simulink model "ACC"  (R2013a)
settings: Solver=ode4  StartTime=0.0  StopTime=100  FixedStep=0.001  MaxStep=0.001  RelTol=1e-3
model workspace (MAT data in the model file):
  m = 1530
  lf = 1.11
  lr = 1.6662
  R_Tire = 0.33
  Iyy_Tire = 0.9
  Pb2Tq_f = 300
  Pb2Tq_r = 150
  Fx_SL = [-1; -0.9; -0.8; -0.7; -0.6; -0.5; -0.4; -0.3; -0.25; -0.2; -0.18; -0.16; -0.14; -0.12; -0.1; -0.08; -0.06; -0.04; -0.02; 0; 0.02; 0.04; 0.06; 0.08; 0.1; 0.12; 0.14; 0.16; 0.18; 0.2; 0.25; 0.3; 0.4; 0.5; 0.6; 0.7; 0.8; 0.9; 1]
  Fx_W = [2105 3995 6120 7900 10100]
  Fx_Data = [-2029.26  -4058.51  -6087.76  -8117.01  -10146.3; -2029.26  -4058.51  -6087.76  -8117.01  -10146.3; -2053.55  -4107.12  -6160.67  -8214.24  -10267.8; -2084.58  -4169.16  -6253.75  -8338.33  -10422.9; -2125.47  -4250.95  -6376.42  -8501.91  -10627.4; -2181.64  -4363.28  -6544.93  -8726.56  -10908.2; -2262.94  -4525.87  -6788.82  -9051.76  -11314.7; -2388.22  -4776.46  -7164.69  -9552.92  -11941.1; -2476.95  -4953.9  -7430.85  -9907.79  -12384.7; -2586.89  -5173.78  -7760.68  -10347.6  -12934.4; -2634.75  -5269.5  -7904.24  -10539  -13173.7; -2680.7  -5361.4  -8042.1  -10722.8  -13403.5; -2717.36  -5434.73  -8152.09  -10869.4  -13586.8; -2729.82  -5459.63  -8189.45  -10919.3  -13649.1; -2689.78  -5379.54  -8069.32  -10759.1  -13448.8; -2548.95  -5097.92  -7646.88  -10195.8  -12744.8; -2240.07  -4480.13  -6720.21  -8960.27  -11200.3; -1701.43  -3402.86  -5104.29  -6805.72  -8507.15; -926.741  -1853.48  -2780.22  -3706.97  -4633.7; 0  0  0  0  0; 926.741  1853.48  2780.22  3706.97  4633.7; 1701.43  3402.86  5104.29  6805.72  8507.15; 2240.07  4480.13  6720.21  8960.27  11200.3; 2548.95  5097.92  7646.88  10195.8  12744.8; 2689.78  5379.54  8069.32  10759.1  13448.8; 2729.82  5459.63  8189.45  10919.3  13649.1; 2717.36  5434.73  8152.09  10869.4  13586.8; 2680.7  5361.4  8042.1  10722.8  13403.5; 2634.75  5269.5  7904.24  10539  13173.7; 2586.89  5173.78  7760.68  10347.6  12934.4; 2476.95  4953.9  7430.85  9907.79  12384.7; 2388.22  4776.46  7164.69  9552.92  11941.1; 2262.94  4525.87  6788.82  9051.76  11314.7; 2181.64  4363.28  6544.93  8726.56  10908.2; 2125.47  4250.95  6376.42  8501.91  10627.4; 2084.58  4169.16  6253.75  8338.33  10422.9; 2053.55  4107.12  6160.67  8214.24  10267.8; 2029.26  4058.51  6087.76  8117.01  10146.3; 2029.26  4058.51  6087.76  8117.01  10146.3]
  g = 9.81
  t2e = 2000
  Fy_Angle = [-20; -16; -14; -12; -10; -9.5; -9; -8.5; -8; -7.5; -7; -6.5; -6; -5.5; -5; -4.5; -4; -3.5; -3; -2.5; -2; -1.5; -1; -0.5; 0; 0.5; 1; 1.5; 2; 2.5; 3; 3.5; 4; 4.5; 5; 5.5; 6; 6.5; 7; 7.5; 8; 8.5; 9; 9.5; 10; 12; 14; 16; 18; 20]
  Fy_W = [1725 3500 6100 6950 9005]
  Fy_Data = [-1523.64 -1531.91 -1546.58 -1574.53 -1631.62 -1653.27 -1678.67 -1707.8 -1740.18 -1775.12 -1810.95 -1845.3 ... (250 elements, 50x5)]
  Cr = 38255
  Cf = 38925
  Izz = 4192
  GearRatio = 17.25
  K = 19
  mu = 0.9
undefined symbols (not defined in the file): sigbuilder_block
libraries: simulink x3
settings Model: Creator=Park  LastModifiedBy=IVDL
settings DataIOCC: LimitDataPoints=off  SignalLoggingSaveFormat=ModelDataLogs
settings OptimizationCC: ExpressionDepthLimit=2147483647
settings DebuggingCC: MultiTaskDSMMsg=warning  MultiTaskCondExecSysMsg=none  FcnCallInpInsideContextMsg=UseLocalSettings  StrictBusMsg=None
settings RTWCC: IncludeERTFirstTime=on
settings GRTTargetCC: CodeReplacementLibrary=None  CombineOutputUpdateFcns=off  CPPClassGenCompliant=on  GRTInterface=on

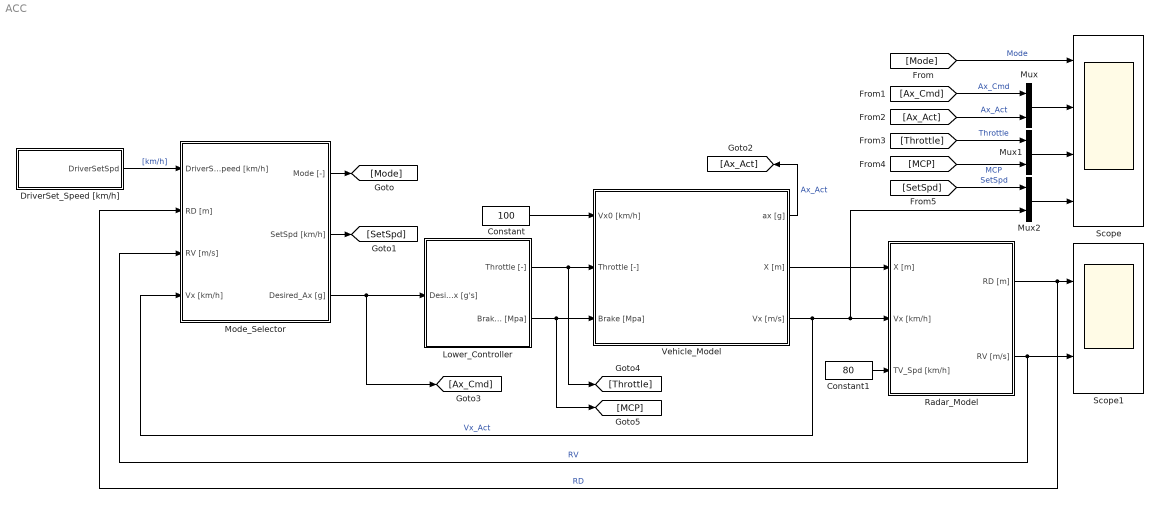
== system ACC ==
  Constant : Constant  Value=100
  Constant1 : Constant  Value=80
  DriverSet_Speed [km/h] : Subsystem  Tag=STV Subsys  LoadFcn=sigbuilder_block('load');  StartFcn=sigbuilder_block('start');  StopFcn=sigbuilder_block('stop');  ClipboardFcn=sigbuilder_block('clipboard');  mask(Sigbuilder block){}
      mask help: Simulink:masks:SigbuilderBlock_MD
      mask init:
      | if ~strcmp(get_param(bdroot(gcbh),'SimulationStatus'),'stopped') tuvar = sigbuilder_block('maskInit'); end
      settings: CopyFcn=sigbuilder_block('copy');  DeleteFcn=sigbuilder_block('delete');  ModelCloseFcn=sigbuilder_block('modelClose');  PreSaveFcn=sigbuilder_block('preSave');  PauseFcn=sigbuilder_block('pause');  ContinueFcn=sigbuilder_block('continue');  NameChangeFcn=sigbuilder_block('namechange');  OpenFcn=sigbuilder_block('open',[361.5 171.75 518.25 401.25 ]);  CloseFcn=sigbuilder_block('close');
      mask Display: plot(0, 0, 100, 100,[2, 2, 32, 32, 2], [68, 8, 8, 68, 68],[32, 2], [38, 38], [32, 19, 2],[53, 60, 44], [32, 17, 17, 2],[16, 16, 31, 31]);txt = getActiveGroup(gcbh);text(2, 100, txt,'verticalAlignment', 'top');
  Lower_Controller : Subsystem
  Mode_Selector : Subsystem
  Mux : Mux  Inputs=2
  Mux1 : Mux  Inputs=2
  Mux2 : Mux  Inputs=2
  Radar_Model : Subsystem
  Scope : Scope  NumInputPorts=4
      settings: ShowLegends=on  TimeRange=100  YMin=0~-0.4~0~30  YMax=1.1~0.4~5~130
  Scope1 : Scope  NumInputPorts=2
      settings: ShowLegends=on  TimeRange=100  YMin=100~-10  YMax=400~6
  Vehicle_Model : Subsystem
  wires:
  Lower_Controller/1(Throttle [-]) -> Vehicle_Model/2(Throttle [-]), [Throttle]
  Lower_Controller/2(Brake [Mpa]) -> Vehicle_Model/3(Brake [Mpa]), [MCP]
  Vehicle_Model/2(X [m]) -> Radar_Model/1(X [m])
  DriverSet_Speed [km/h]/1(DriverSetSpd) -> Mode_Selector/1(DriverSet_Speed [km/h])  "[km/h]"
  Constant/1 -> Vehicle_Model/1(Vx0 [km/h])
  Radar_Model/1(RD [m]) -> Mode_Selector/2(RD [m]), Scope1/1  "RD"
  Radar_Model/2(RV [m/s]) -> Mode_Selector/3(RV [m/s]), Scope1/2  "RV"
  Constant1/1 -> Radar_Model/3(TV_Spd [km/h])
  Mode_Selector/1(Mode [-]) -> [Mode]
  Mode_Selector/2(SetSpd [km/h]) -> [SetSpd]
  Vehicle_Model/1(ax [g]) -> [Ax_Act]  "Ax_Act"
  [Mode] -> Scope/1  "Mode"
  Mux/1 -> Scope/2
  [Ax_Cmd] -> Mux/1  "Ax_Cmd"
  [Ax_Act] -> Mux/2  "Ax_Act"
  Mux1/1 -> Scope/3
  [MCP] -> Mux1/2  "MCP"
  [Throttle] -> Mux1/1  "Throttle"
  Mux2/1 -> Scope/4
  [SetSpd] -> Mux2/1  "SetSpd"
  Vehicle_Model/3(Vx [m/s]) -> Mode_Selector/4(Vx [km/h]), Mux2/2, Radar_Model/2(Vx [km/h])  "Vx_Act"
  Mode_Selector/3(Desired_Ax [g]) -> [Ax_Cmd], Lower_Controller/1(Desired_Ax [g's])

== system ACC/DriverSet_Speed [km//h] ==
  Demux : Demux  Tag=STV Demux  Outputs=1
  FromWs : FromWorkspace  Tag=STV FromWs  VariableName=tuvar  SampleTime=0
      SigBuilderData=|
      | common.afterFinalStr = 'Extrapolate'
      | common.sampleTime = 0
      | dataSet.timeRange = [0 100]
      | dataSet.name = 'Group 1'
      | sbobj.Groups.Name = 'Group 1'
      | sbobj.Groups.Signals.Name = 'DriverSetSpd'
      | sbobj.Groups.Signals.XData = [0 25 25 80 80 100]
      | sbobj.Groups.Signals.YData = [70 70 110 110 60 60]
      | sbobj.Groups.TimeRange = [0 100]
  DriverSetSpd : Outport  Tag=STV Outport
  wires:
  FromWs/1 -> Demux/1
  Demux/1 -> DriverSetSpd/1

== system ACC/Lower_Controller ==
  Desired_Ax [g's] : Inport
  Brake_Controller : Subsystem  RequirementInfo="{}  %GIDa_30b132b4_0fb0_4af6_85f4_ad121309f217"
  Throttle_Controller : Subsystem  RequirementInfo="{}  %GIDa_10e5c59a_a8ca_4e4d_9e23_d4de8c8e8e1e"
  Throttle [-] : Outport
  Brake [Mpa] : Outport  Port=2
  wires:
  Desired_Ax [g's]/1 -> Throttle_Controller/1(Desired_Ax [g's]), Brake_Controller/1(Desired_Ax [g's])
  Throttle_Controller/1(Throttle [-]) -> Throttle [-]/1
  Brake_Controller/1(Brake [Mpa]) -> Brake [Mpa]/1

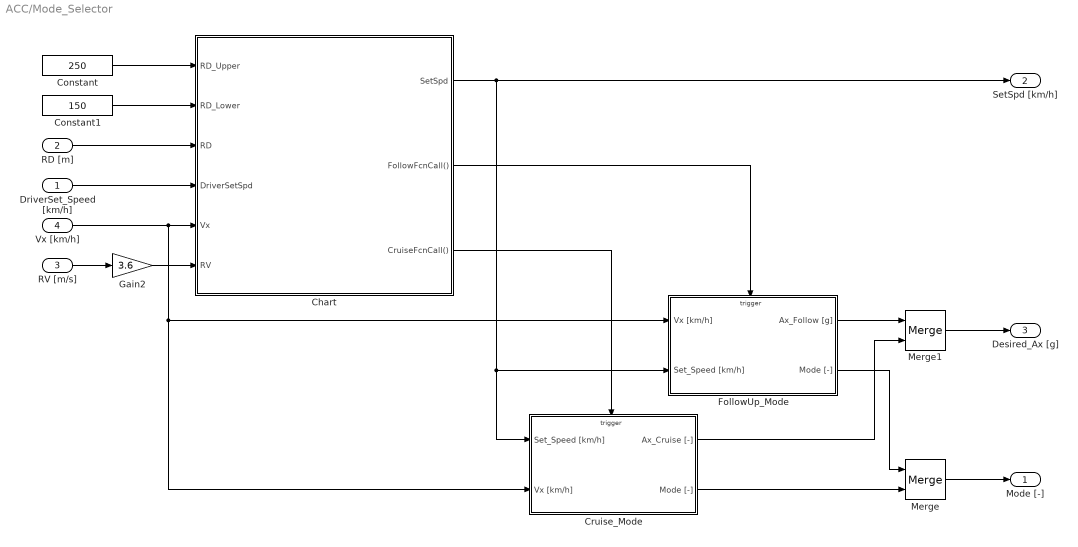
== system ACC/Mode_Selector ==
  DriverSet_Speed [km/h] : Inport
  RD [m] : Inport  Port=2
  RV [m/s] : Inport  Port=3
  Vx [km/h] : Inport  Port=4
  Chart : Stateflow chart  TreatAsAtomicUnit=on
  Constant : Constant  Value=250
  Constant1 : Constant  Value=150
  Cruise_Mode : Subsystem
  FollowUp_Mode : Subsystem
  Gain2 : Gain  Gain=3.6
  Merge : Merge
  Merge1 : Merge
  Mode [-] : Outport
  SetSpd [km/h] : Outport  Port=2
  Desired_Ax [g] : Outport  Port=3
  wires:
  Constant1/1 -> Chart/2(RD_Lower)
  Constant/1 -> Chart/1(RD_Upper)
  RV [m/s]/1 -> Gain2/1
  DriverSet_Speed [km/h]/1 -> Chart/4(DriverSetSpd)
  RD [m]/1 -> Chart/3(RD)
  Vx [km/h]/1 -> Cruise_Mode/2(Vx [km/h]), FollowUp_Mode/1(Vx [km/h]), Chart/5(Vx)
  Gain2/1 -> Chart/6(RV)
  Chart/2(FollowFcnCall()) -> FollowUp_Mode/Trigger
  Chart/3(CruiseFcnCall()) -> Cruise_Mode/Trigger
  Merge1/1 -> Desired_Ax [g]/1
  FollowUp_Mode/1(Ax_Follow [g]) -> Merge1/1
  Cruise_Mode/1(Ax_Cruise [-]) -> Merge1/2
  FollowUp_Mode/2(Mode [-]) -> Merge/1
  Cruise_Mode/2(Mode [-]) -> Merge/2
  Merge/1 -> Mode [-]/1
  Chart/1(SetSpd) -> SetSpd [km/h]/1, FollowUp_Mode/2(Set_Speed [km/h]), Cruise_Mode/1(Set_Speed [km/h])

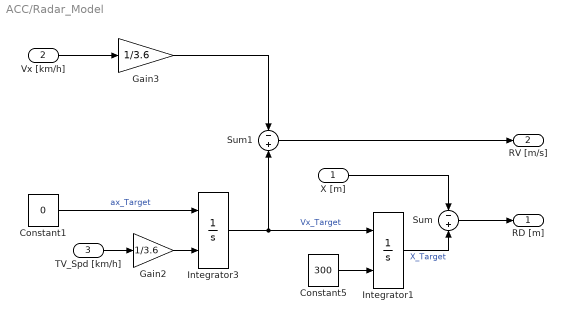
== system ACC/Radar_Model ==
  X [m] : Inport
  Vx [km/h] : Inport  Port=2
  TV_Spd [km/h] : Inport  Port=3
  Constant1 : Constant  Value=0
  Constant5 : Constant  Value=300
  Gain2 : Gain  Gain=1/3.6
  Gain3 : Gain  Gain=1/3.6
  Integrator1 : Integrator  InitialConditionSource=external  InitialCondition=500
  Integrator3 : Integrator  InitialConditionSource=external  InitialCondition=80  LimitOutput=on  LowerSaturationLimit=0
  Sum : Sum  Inputs=-+
  Sum1 : Sum  Inputs=-+
  RD [m] : Outport
  RV [m/s] : Outport  Port=2
  wires:
  TV_Spd [km/h]/1 -> Gain2/1
  Constant1/1 -> Integrator3/1  "ax_Target"
  Integrator3/1 -> Integrator1/1, Sum1/2  "Vx_Target"
  Integrator1/1 -> Sum/2  "X_Target"
  Constant5/1 -> Integrator1/2
  Sum/1 -> RD [m]/1
  X [m]/1 -> Sum/1
  Vx [km/h]/1 -> Gain3/1
  Sum1/1 -> RV [m/s]/1
  Gain2/1 -> Integrator3/2
  Gain3/1 -> Sum1/1

== system ACC/Vehicle_Model ==
  Vx0 [km/h] : Inport
  Throttle [-] : Inport  Port=2
  Brake [Mpa] : Inport  Port=3
  Gain1 : Gain  Gain=1/9.81
  Gain2 : Gain  Gain=3.6
  SWA [deg] : Constant  Value=0
  Vehicle_Model : Subsystem
  ax [g] : Outport
  X [m] : Outport  Port=2
  Vx [m/s] : Outport  Port=3
  wires:
  Vx0 [km/h]/1 -> Vehicle_Model/1(Vx0 [km/h])
  SWA [deg]/1 -> Vehicle_Model/2(SWA [deg])
  Vehicle_Model/5(Vx [m/s]) -> Gain2/1
  Vehicle_Model/6(ax [m/s^2]) -> Gain1/1
  Brake [Mpa]/1 -> Vehicle_Model/4(Brake [Mpa])
  Throttle [-]/1 -> Vehicle_Model/3(Throttle [-])
  Vehicle_Model/1(X [m]) -> X [m]/1
  Gain2/1 -> Vx [m/s]/1
  Gain1/1 -> ax [g]/1

== system ACC/Lower_Controller/Brake_Controller ==
  Desired_Ax [g's] : Inport
  Compare To Zero : simulink/Logic and Bit Operations/Compare To Zero  relop=<=  OutDataTypeStr=boolean
  Data Type Conversion : DataTypeConversion  OutDataTypeStr=double
  Gain : Gain  Gain=-1
  Gain1 : Gain  Gain=0.05
  Gain2 : Gain  Gain=12
  Integrator : Integrator  ExternalReset=rising
  Saturation : Saturate  UpperLimit=4  LowerLimit=0
  Sum : Sum
  Brake [Mpa] : Outport
  wires:
  Gain/1 -> Gain2/1, Gain1/1, Compare To Zero/1
  Saturation/1 -> Brake [Mpa]/1
  Sum/1 -> Saturation/1
  Desired_Ax [g's]/1 -> Gain/1
  Gain2/1 -> Sum/1
  Compare To Zero/1 -> Data Type Conversion/1
  Integrator/1 -> Sum/2
  Gain1/1 -> Integrator/1
  Data Type Conversion/1 -> Integrator/2

== system ACC/Lower_Controller/Throttle_Controller ==
  Desired_Ax [g's] : Inport
  Compare To Zero : simulink/Logic and Bit Operations/Compare To Zero  relop=<=  OutDataTypeStr=boolean
  Data Type Conversion : DataTypeConversion  OutDataTypeStr=double
  Gain1 : Gain  Gain=0.5
  Gain2 : Gain  Gain=7
  Integrator : Integrator  ExternalReset=rising
  Saturation : Saturate  UpperLimit=0.7  LowerLimit=0
  Sum : Sum
  Throttle [-] : Outport
  wires:
  Saturation/1 -> Throttle [-]/1
  Sum/1 -> Saturation/1
  Desired_Ax [g's]/1 -> Gain2/1, Gain1/1, Compare To Zero/1
  Gain2/1 -> Sum/1
  Integrator/1 -> Sum/2
  Data Type Conversion/1 -> Integrator/2
  Gain1/1 -> Integrator/1
  Compare To Zero/1 -> Data Type Conversion/1

== system ACC/Mode_Selector/Cruise_Mode ==
  Set_Speed [km/h] : Inport
  Vx [km/h] : Inport  Port=2
  function : TriggerPort  TriggerType=function-call
  Divide : Product  Inputs=/*
  Gain : Gain  Gain=1.2
  Mode1 : Constant  Value=0
  Saturation : Saturate  UpperLimit=0.3  LowerLimit=-0.3
  Sum : Sum  Inputs=|+-
  Ax_Cruise [-] : Outport
  Mode [-] : Outport  Port=2
  wires:
  Vx [km/h]/1 -> Sum/2
  Mode1/1 -> Mode [-]/1
  Saturation/1 -> Ax_Cruise [-]/1
  Divide/1 -> Gain/1  "Normalized_Vx"
  Sum/1 -> Divide/2
  Set_Speed [km/h]/1 -> Divide/1, Sum/1
  Gain/1 -> Saturation/1

== system ACC/Mode_Selector/FollowUp_Mode ==
  Vx [km/h] : Inport
  Set_Speed [km/h] : Inport  Port=2
  function : TriggerPort  TriggerType=function-call
  Divide : Product  Inputs=/*
  Gain : Gain  Gain=2
  Mode1 : Constant
  Saturation1 : Saturate  UpperLimit=0.4  LowerLimit=-0.4
  Sum1 : Sum  Inputs=|+-
  Ax_Follow [g] : Outport
  Mode [-] : Outport  Port=2
  wires:
  Vx [km/h]/1 -> Sum1/2
  Set_Speed [km/h]/1 -> Sum1/1, Divide/1
  Saturation1/1 -> Ax_Follow [g]/1
  Divide/1 -> Gain/1  "Normalized_Vx"
  Sum1/1 -> Divide/2
  Mode1/1 -> Mode [-]/1
  Gain/1 -> Saturation1/1

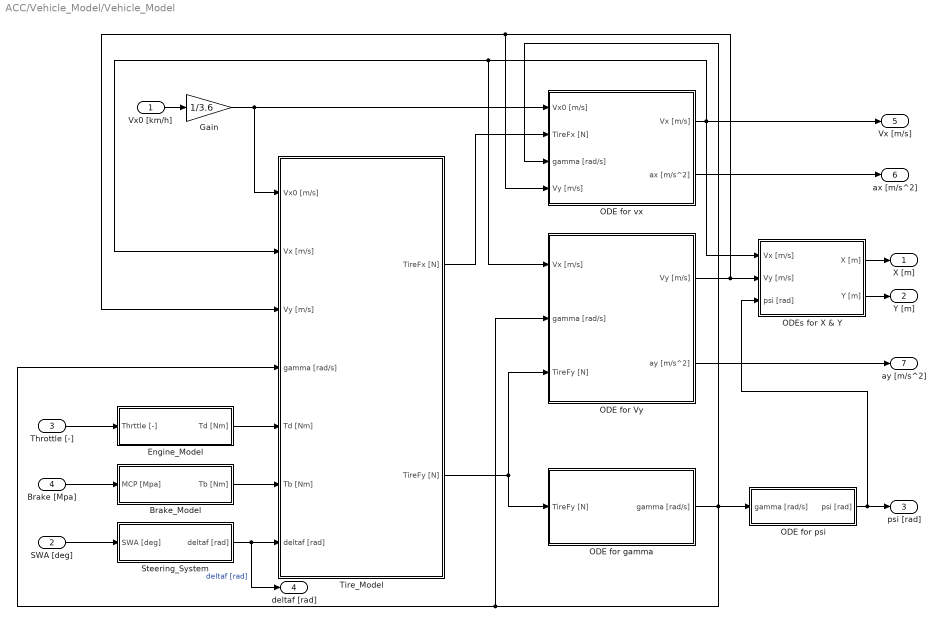
== system ACC/Vehicle_Model/Vehicle_Model ==
  Vx0 [km/h] : Inport
  SWA [deg] : Inport  Port=2
  Throttle [-] : Inport  Port=3
  Brake [Mpa] : Inport  Port=4
  Brake_Model : Subsystem
  Engine_Model : Subsystem
  Gain : Gain  Gain=1/3.6
  ODE for Vy : Subsystem
  ODE for gamma : Subsystem
  ODE for psi : Subsystem
  ODE for vx : Subsystem
  ODEs for X & Y : Subsystem
  Steering_System : Subsystem
  Tire_Model : Subsystem
  X [m] : Outport
  Y [m] : Outport  Port=2
  psi [rad] : Outport  Port=3
  deltaf [rad] : Outport  Port=4
  Vx [m/s] : Outport  Port=5
  ax [m/s^2] : Outport  Port=6
  ay [m/s^2] : Outport  Port=7
  wires:
  Vx0 [km/h]/1 -> Gain/1
  SWA [deg]/1 -> Steering_System/1(SWA [deg])
  Gain/1 -> ODE for vx/1(Vx0 [m/s]), Tire_Model/1(Vx0 [m/s])
  Engine_Model/1(Td [Nm]) -> Tire_Model/5(Td [Nm])
  Brake_Model/1(Tb [Nm]) -> Tire_Model/6(Tb [Nm])
  Brake [Mpa]/1 -> Brake_Model/1(MCP [Mpa])
  Throttle [-]/1 -> Engine_Model/1(Thrttle [-])
  Tire_Model/1(TireFx [N]) -> ODE for vx/2(TireFx [N])
  Steering_System/1(deltaf [rad]) -> deltaf [rad]/1, Tire_Model/7(deltaf [rad])  "deltaf [rad]"
  ODE for vx/1(Vx [m/s]) -> Vx [m/s]/1, ODEs for X & Y/1(Vx [m/s]), ODE for Vy/1(Vx [m/s]), Tire_Model/2(Vx [m/s])
  Tire_Model/2(TireFy [N]) -> ODE for Vy/3(TireFy [N]), ODE for gamma/1(TireFy [N])
  ODE for gamma/1(gamma [rad/s]) -> ODE for vx/3(gamma [rad/s]), ODE for psi/1(gamma [rad/s]), Tire_Model/4(gamma [rad/s]), ODE for Vy/2(gamma [rad/s])
  ODE for Vy/1(Vy [m/s]) -> ODE for vx/4(Vy [m/s]), Tire_Model/3(Vy [m/s]), ODEs for X & Y/2(Vy [m/s])
  ODE for psi/1(psi [rad]) -> psi [rad]/1, ODEs for X & Y/3(psi [rad])
  ODEs for X & Y/1(X [m]) -> X [m]/1
  ODEs for X & Y/2(Y [m]) -> Y [m]/1
  ODE for vx/2(ax [m/s^2]) -> ax [m/s^2]/1
  ODE for Vy/2(ay [m/s^2]) -> ay [m/s^2]/1

== system ACC/Vehicle_Model/Vehicle_Model/Brake_Model ==
  MCP [Mpa] : Inport
  Gain : Gain  Gain=2*Pb2Tq_f
  Gain1 : Gain  Gain=2*Pb2Tq_r
  Mux : Mux  Inputs=2
  Transfer Fcn : TransferFcn  Denominator=[0.06 1]
  Transfer Fcn1 : TransferFcn  Denominator=[0.06 1]
  Tb [Nm] : Outport
  wires:
  Gain/1 -> Transfer Fcn/1  "Tb_f [Nm]"
  Gain1/1 -> Transfer Fcn1/1  "Tb_r [Nm]"
  MCP [Mpa]/1 -> Gain1/1, Gain/1
  Mux/1 -> Tb [Nm]/1
  Transfer Fcn/1 -> Mux/1
  Transfer Fcn1/1 -> Mux/2

== system ACC/Vehicle_Model/Vehicle_Model/Engine_Model ==
  Thrttle [-] : Inport
  Gain : Gain  Gain=t2e
  Transfer Fcn : TransferFcn  Numerator=[100]  Denominator=[1 2*0.5*10 100]
  Td [Nm] : Outport
  wires:
  Thrttle [-]/1 -> Gain/1
  Gain/1 -> Transfer Fcn/1
  Transfer Fcn/1 -> Td [Nm]/1

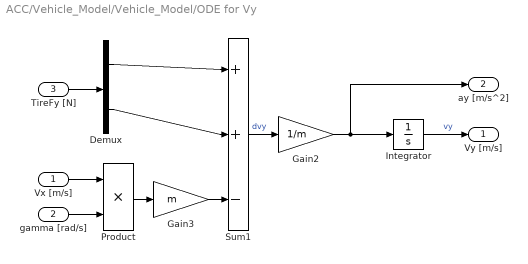
== system ACC/Vehicle_Model/Vehicle_Model/ODE for Vy ==
  Vx [m/s] : Inport
  gamma [rad/s] : Inport  Port=2
  TireFy [N] : Inport  Port=3
  Demux : Demux  Outputs=2
  Gain2 : Gain  Gain=1/m
  Gain3 : Gain  Gain=m
  Integrator : Integrator
  Product : Product  RndMeth=Zero
  Sum1 : Sum  Inputs=++|-
  Vy [m/s] : Outport
  ay [m/s^2] : Outport  Port=2
  wires:
  Demux/1 -> Sum1/1
  Demux/2 -> Sum1/2
  Sum1/1 -> Gain2/1  "dvy"
  Product/1 -> Gain3/1
  Integrator/1 -> Vy [m/s]/1  "vy"
  Vx [m/s]/1 -> Product/1
  gamma [rad/s]/1 -> Product/2
  TireFy [N]/1 -> Demux/1
  Gain3/1 -> Sum1/3
  Gain2/1 -> ay [m/s^2]/1, Integrator/1

== system ACC/Vehicle_Model/Vehicle_Model/ODE for gamma ==
  TireFy [N] : Inport
  Demux : Demux  Outputs=2
  Gain4 : Gain  Gain=1/Izz
  Gain5 : Gain  Gain=lf
  Gain6 : Gain  Gain=lr
  Integrator2 : Integrator
  Sum2 : Sum  Inputs=+-
  gamma [rad/s] : Outport
  wires:
  Sum2/1 -> Gain4/1
  Gain4/1 -> Integrator2/1
  Gain5/1 -> Sum2/1
  Gain6/1 -> Sum2/2
  Demux/1 -> Gain5/1
  Integrator2/1 -> gamma [rad/s]/1  "gamma"
  Demux/2 -> Gain6/1
  TireFy [N]/1 -> Demux/1

== system ACC/Vehicle_Model/Vehicle_Model/ODE for psi ==
  gamma [rad/s] : Inport
  Integrator : Integrator  ContinuousStateAttributes='psi'
  psi [rad] : Outport
  wires:
  Integrator/1 -> psi [rad]/1
  gamma [rad/s]/1 -> Integrator/1  "dpsi"

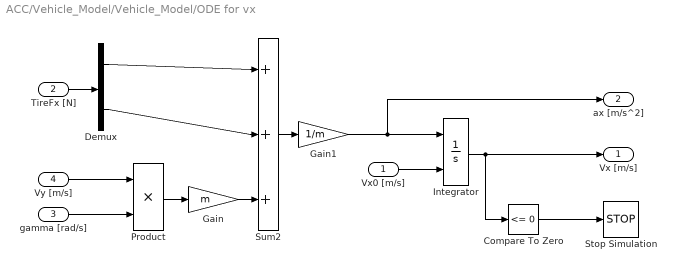
== system ACC/Vehicle_Model/Vehicle_Model/ODE for vx ==
  Vx0 [m/s] : Inport
  TireFx [N] : Inport  Port=2
  gamma [rad/s] : Inport  Port=3
  Vy [m/s] : Inport  Port=4
  Compare To Zero : simulink/Logic and Bit Operations/Compare To Zero  relop=<=  OutDataTypeStr=boolean
  Demux : Demux  Outputs=2
  Gain : Gain  Gain=m
  Gain1 : Gain  Gain=1/m
  Integrator : Integrator  InitialConditionSource=external
  Product : Product  RndMeth=Zero
  Stop Simulation : Stop
  Sum2 : Sum  Inputs=++|+
  Vx [m/s] : Outport
  ax [m/s^2] : Outport  Port=2
  wires:
  Vx0 [m/s]/1 -> Integrator/2
  Integrator/1 -> Compare To Zero/1, Vx [m/s]/1
  TireFx [N]/1 -> Demux/1
  Demux/1 -> Sum2/1
  Demux/2 -> Sum2/2
  Vy [m/s]/1 -> Product/1
  gamma [rad/s]/1 -> Product/2
  Sum2/1 -> Gain1/1
  Product/1 -> Gain/1
  Gain/1 -> Sum2/3
  Compare To Zero/1 -> Stop Simulation/1
  Gain1/1 -> ax [m/s^2]/1, Integrator/1

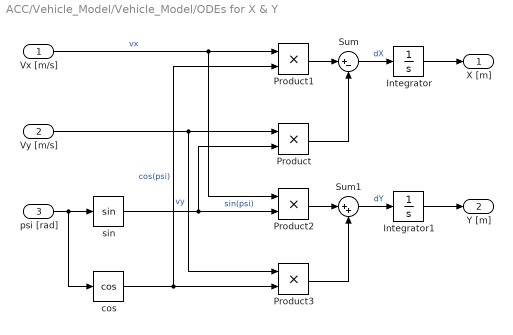
== system ACC/Vehicle_Model/Vehicle_Model/ODEs for X & Y ==
  Vx [m/s] : Inport
  Vy [m/s] : Inport  Port=2
  psi [rad] : Inport  Port=3
  Integrator : Integrator  ContinuousStateAttributes='X'
  Integrator1 : Integrator  ContinuousStateAttributes='Y'
  Product{,1..3} (4 alike) : Product  RndMeth=Zero
  Sum : Sum  Inputs=|+-
  Sum1 : Sum  Inputs=|++
  cos : Trigonometry  Operator=cos
  sin : Trigonometry
  X [m] : Outport
  Y [m] : Outport  Port=2
  wires:
  psi [rad]/1 -> sin/1, cos/1
  sin/1 -> Product/2, Product2/2  "sin(psi)"
  Vy [m/s]/1 -> Product/1, Product3/1  "vy"
  Vx [m/s]/1 -> Product1/1, Product2/1  "vx"
  cos/1 -> Product1/2, Product3/2  "cos(psi)"
  Product1/1 -> Sum/1
  Product/1 -> Sum/2
  Sum/1 -> Integrator/1  "dX"
  Product2/1 -> Sum1/1
  Product3/1 -> Sum1/2
  Sum1/1 -> Integrator1/1  "dY"
  Integrator/1 -> X [m]/1
  Integrator1/1 -> Y [m]/1

== system ACC/Vehicle_Model/Vehicle_Model/Steering_System ==
  SWA [deg] : Inport
  Gain : Gain  Gain=1/GearRatio
  Gain5 : Gain  Gain=pi/180
  Saturation : Saturate  UpperLimit=540  LowerLimit=-540
  deltaf [rad] : Outport
  wires:
  Gain/1 -> Gain5/1
  Gain5/1 -> deltaf [rad]/1
  SWA [deg]/1 -> Saturation/1
  Saturation/1 -> Gain/1

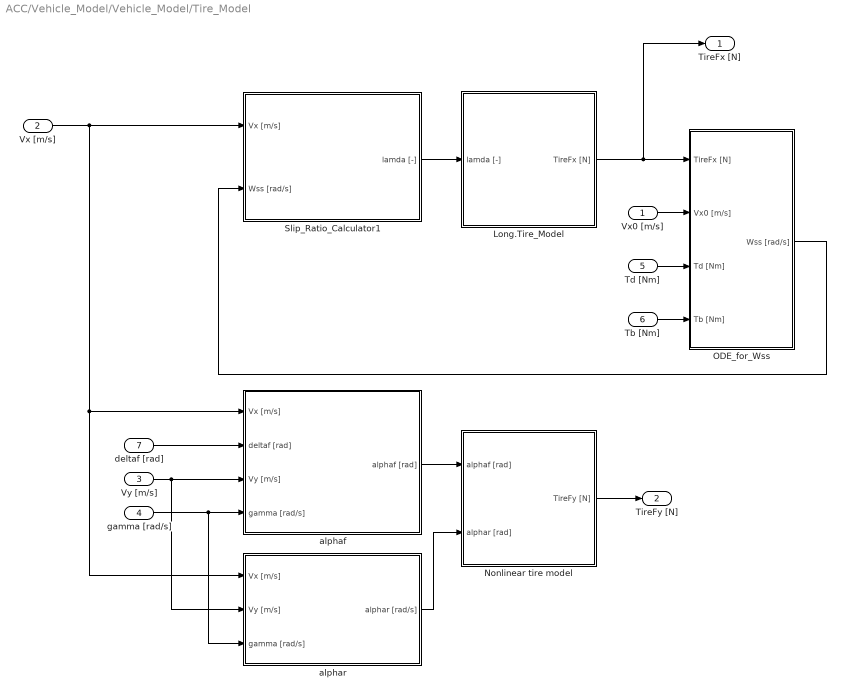
== system ACC/Vehicle_Model/Vehicle_Model/Tire_Model ==
  Vx0 [m/s] : Inport
  Vx [m/s] : Inport  Port=2
  Vy [m/s] : Inport  Port=3
  gamma [rad/s] : Inport  Port=4
  Td [Nm] : Inport  Port=5
  Tb [Nm] : Inport  Port=6
  deltaf [rad] : Inport  Port=7
  Long.Tire_Model : Subsystem
  Nonlinear tire model : Subsystem
  ODE_for_Wss : Subsystem
  Slip_Ratio_Calculator1 : Subsystem
  alphaf : Subsystem
  alphar : Subsystem
  TireFx [N] : Outport
  TireFy [N] : Outport  Port=2
  wires:
  Long.Tire_Model/1(TireFx [N]) -> TireFx [N]/1, ODE_for_Wss/1(TireFx [N])
  Slip_Ratio_Calculator1/1(lamda [-]) -> Long.Tire_Model/1(lamda [-])
  Vx [m/s]/1 -> Slip_Ratio_Calculator1/1(Vx [m/s]), alphar/1(Vx [m/s]), alphaf/1(Vx [m/s])
  Vx0 [m/s]/1 -> ODE_for_Wss/2(Vx0 [m/s])
  Td [Nm]/1 -> ODE_for_Wss/3(Td [Nm])
  Tb [Nm]/1 -> ODE_for_Wss/4(Tb [Nm])
  ODE_for_Wss/1(Wss [rad/s]) -> Slip_Ratio_Calculator1/2(Wss [rad/s])
  alphaf/1(alphaf [rad]) -> Nonlinear tire model/1(alphaf [rad])
  alphar/1(alphar [rad/s]) -> Nonlinear tire model/2(alphar [rad])
  deltaf [rad]/1 -> alphaf/2(deltaf [rad])
  Vy [m/s]/1 -> alphaf/3(Vy [m/s]), alphar/2(Vy [m/s])
  gamma [rad/s]/1 -> alphar/3(gamma [rad/s]), alphaf/4(gamma [rad/s])
  Nonlinear tire model/1(TireFy [N]) -> TireFy [N]/1

== system ACC/Vehicle_Model/Vehicle_Model/Tire_Model/Long.Tire_Model ==
  lamda [-] : Inport
  Demux : Demux  Outputs=2
  Fx_f_Calculator : Subsystem
  Fx_r_Calculator : Subsystem
  Mux : Mux  Inputs=2
  TireFx [N] : Outport
  wires:
  lamda [-]/1 -> Demux/1
  Demux/1 -> Fx_f_Calculator/1(lamda_f [-])
  Demux/2 -> Fx_r_Calculator/1(lamda_r [-])
  Fx_f_Calculator/1(TireFx _f [N]) -> Mux/1
  Fx_r_Calculator/1(TireFx _r [N]) -> Mux/2
  Mux/1 -> TireFx [N]/1

== system ACC/Vehicle_Model/Vehicle_Model/Tire_Model/Nonlinear tire model ==
  alphaf [rad] : Inport
  alphar [rad] : Inport  Port=2
  Gain : Gain  Gain=-2*Cf*mu/K
  Gain1 : Gain  Gain=-2*Cr*mu/K
  Gain2 : Gain  Gain=K/mu
  Gain3 : Gain  Gain=K/mu
  Mux : Mux  Inputs=2
  atan : Trigonometry  Operator=atan
  atan1 : Trigonometry  Operator=atan
  TireFy [N] : Outport
  wires:
  Mux/1 -> TireFy [N]/1
  Gain2/1 -> atan/1
  atan/1 -> Gain/1
  Gain3/1 -> atan1/1
  atan1/1 -> Gain1/1
  alphaf [rad]/1 -> Gain2/1
  alphar [rad]/1 -> Gain3/1
  Gain1/1 -> Mux/2
  Gain/1 -> Mux/1

== system ACC/Vehicle_Model/Vehicle_Model/Tire_Model/ODE_for_Wss ==
  TireFx [N] : Inport
  Vx0 [m/s] : Inport  Port=2
  Td [Nm] : Inport  Port=3
  Tb [Nm] : Inport  Port=4
  Demux : Demux  Outputs=2
  Demux1 : Demux  Outputs=2
  Mux : Mux  Inputs=2
  ODE_for_Wss_f : Subsystem
  ODE_for_Wss_r : Subsystem
  Wss [rad/s] : Outport
  wires:
  Demux1/1 -> ODE_for_Wss_f/3(TireFx _f [N])  "TireFx _f [N]"
  Td [Nm]/1 -> ODE_for_Wss_f/1(Td_f [Nm])
  Vx0 [m/s]/1 -> ODE_for_Wss_r/1(Vx0 [m/s]), ODE_for_Wss_f/2(Vx0 [m/s])
  Tb [Nm]/1 -> Demux/1
  Demux/1 -> ODE_for_Wss_f/4(Tb_f [Nm])
  Demux/2 -> ODE_for_Wss_r/3(Tb_r [Nm])
  TireFx [N]/1 -> Demux1/1
  Demux1/2 -> ODE_for_Wss_r/2(TireFx _r [N])  "TireFx _r [N]"
  ODE_for_Wss_f/1(Wss_f [rad/s]) -> Mux/1
  ODE_for_Wss_r/1(Wss_r [rad/s]) -> Mux/2
  Mux/1 -> Wss [rad/s]/1

== system ACC/Vehicle_Model/Vehicle_Model/Tire_Model/Slip_Ratio_Calculator1 ==
  Vx [m/s] : Inport
  Wss [rad/s] : Inport  Port=2
  Demux : Demux  Outputs=2
  Mux : Mux  Inputs=2
  lamda_f_Calculator : Subsystem
  lamda_r_Calculator : Subsystem
  lamda [-] : Outport
  wires:
  Vx [m/s]/1 -> lamda_f_Calculator/2(Vx [m/s]), lamda_r_Calculator/2(Vx [m/s])
  lamda_f_Calculator/1(lamda_f [-]) -> Mux/1  "lamda_f [-]"
  lamda_r_Calculator/1(lamda_f [-]) -> Mux/2  "lamda_r [-]"
  Mux/1 -> lamda [-]/1
  Wss [rad/s]/1 -> Demux/1
  Demux/1 -> lamda_f_Calculator/1(Wss_f [rad/s])  "Wss_f [rad/s]"
  Demux/2 -> lamda_r_Calculator/1(Wss_r [rad/s])  "Wss_r [rad/s]"

== system ACC/Vehicle_Model/Vehicle_Model/Tire_Model/alphaf ==
  Vx [m/s] : Inport
  deltaf [rad] : Inport  Port=2
  Vy [m/s] : Inport  Port=3
  gamma [rad/s] : Inport  Port=4
  Divide : Product  Inputs=*/
  Gain : Gain  Gain=lf
  Sum : Sum  Inputs=++|
  Sum1 : Sum  Inputs=|+-
  Trigonometric Function : Trigonometry  Operator=atan
  alphaf [rad] : Outport
  wires:
  gamma [rad/s]/1 -> Gain/1
  Vy [m/s]/1 -> Sum/1
  Gain/1 -> Sum/2
  Sum/1 -> Divide/1
  Vx [m/s]/1 -> Divide/2
  Divide/1 -> Trigonometric Function/1
  Trigonometric Function/1 -> Sum1/1
  deltaf [rad]/1 -> Sum1/2
  Sum1/1 -> alphaf [rad]/1

== system ACC/Vehicle_Model/Vehicle_Model/Tire_Model/alphar ==
  Vx [m/s] : Inport
  Vy [m/s] : Inport  Port=2
  gamma [rad/s] : Inport  Port=3
  Divide : Product  Inputs=*/
  Gain : Gain  Gain=lr
  Sum : Sum  Inputs=+-|
  Trigonometric Function : Trigonometry  Operator=atan
  alphar [rad/s] : Outport
  wires:
  Trigonometric Function/1 -> alphar [rad/s]/1
  Divide/1 -> Trigonometric Function/1
  Vx [m/s]/1 -> Divide/2
  Sum/1 -> Divide/1
  Gain/1 -> Sum/2
  Vy [m/s]/1 -> Sum/1
  gamma [rad/s]/1 -> Gain/1

== system ACC/Vehicle_Model/Vehicle_Model/Tire_Model/Long.Tire_Model/Fx_f_Calculator ==
  lamda_f [-] : Inport
  Constant : Constant  Value=m*9.81
  Fx_Table_fl : Lookup2D  RowIndex=Fx_SL  ColumnIndex=Fx_W  Table=Fx_Data  SaturateOnIntegerOverflow=on
  Gain : Gain  Gain=lr / (lf+lr)
  Gain1 : Gain  Gain=2
  Gain4 : Gain  Gain=0.5
  TireFx _f [N] : Outport
  wires:
  Gain1/1 -> TireFx _f [N]/1
  lamda_f [-]/1 -> Fx_Table_fl/1
  Constant/1 -> Gain/1
  Gain/1 -> Gain4/1
  Gain4/1 -> Fx_Table_fl/2  "Wf [N]"
  Fx_Table_fl/1 -> Gain1/1

== system ACC/Vehicle_Model/Vehicle_Model/Tire_Model/Long.Tire_Model/Fx_r_Calculator ==
  lamda_r [-] : Inport
  Constant1 : Constant  Value=m*9.81
  Fx_Table_fl1 : Lookup2D  RowIndex=Fx_SL  ColumnIndex=Fx_W  Table=Fx_Data  SaturateOnIntegerOverflow=on
  Gain2 : Gain  Gain=lf / (lf+lr)
  Gain3 : Gain  Gain=2
  Gain5 : Gain  Gain=0.5
  TireFx _r [N] : Outport
  wires:
  lamda_r [-]/1 -> Fx_Table_fl1/1
  Constant1/1 -> Gain2/1
  Fx_Table_fl1/1 -> Gain3/1
  Gain2/1 -> Gain5/1
  Gain5/1 -> Fx_Table_fl1/2  "Wr [N]"
  Gain3/1 -> TireFx _r [N]/1

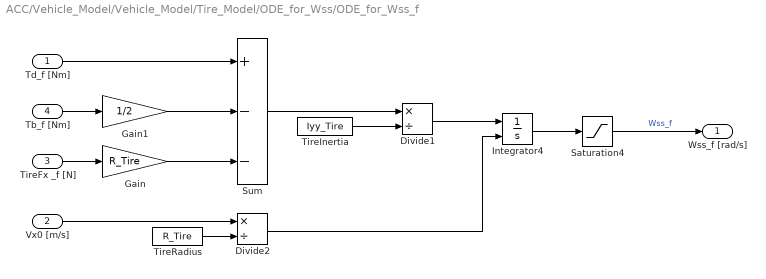
== system ACC/Vehicle_Model/Vehicle_Model/Tire_Model/ODE_for_Wss/ODE_for_Wss_f ==
  Td_f [Nm] : Inport
  Vx0 [m/s] : Inport  Port=2
  TireFx _f [N] : Inport  Port=3
  Tb_f [Nm] : Inport  Port=4
  Divide1 : Product  Inputs=*/
  Divide2 : Product  Inputs=*/
  Gain : Gain  Gain=R_Tire
  Gain1 : Gain  Gain=1/2
  Integrator4 : Integrator  InitialConditionSource=external
  Saturation4 : Saturate  UpperLimit=255  LowerLimit=0
  Sum : Sum  Inputs=+--
  TireInertia : Constant  Value=Iyy_Tire
  TireRadius : Constant  Value=R_Tire
  Wss_f [rad/s] : Outport
  wires:
  Gain/1 -> Sum/3
  Td_f [Nm]/1 -> Sum/1
  Tb_f [Nm]/1 -> Gain1/1
  TireFx _f [N]/1 -> Gain/1
  Sum/1 -> Divide1/1
  TireInertia/1 -> Divide1/2
  Divide1/1 -> Integrator4/1
  TireRadius/1 -> Divide2/2
  Vx0 [m/s]/1 -> Divide2/1
  Divide2/1 -> Integrator4/2
  Integrator4/1 -> Saturation4/1
  Saturation4/1 -> Wss_f [rad/s]/1  "Wss_f"
  Gain1/1 -> Sum/2

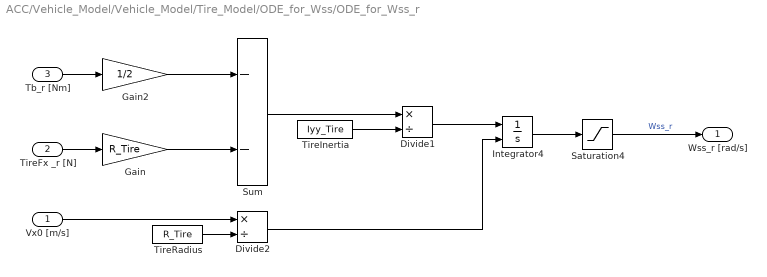
== system ACC/Vehicle_Model/Vehicle_Model/Tire_Model/ODE_for_Wss/ODE_for_Wss_r ==
  Vx0 [m/s] : Inport
  TireFx _r [N] : Inport  Port=2
  Tb_r [Nm] : Inport  Port=3
  Divide1 : Product  Inputs=*/
  Divide2 : Product  Inputs=*/
  Gain : Gain  Gain=R_Tire
  Gain2 : Gain  Gain=1/2
  Integrator4 : Integrator  InitialConditionSource=external
  Saturation4 : Saturate  UpperLimit=255  LowerLimit=0
  Sum : Sum  Inputs=--
  TireInertia : Constant  Value=Iyy_Tire
  TireRadius : Constant  Value=R_Tire
  Wss_r [rad/s] : Outport
  wires:
  Saturation4/1 -> Wss_r [rad/s]/1  "Wss_r"
  Integrator4/1 -> Saturation4/1
  Divide2/1 -> Integrator4/2
  Vx0 [m/s]/1 -> Divide2/1
  TireRadius/1 -> Divide2/2
  Divide1/1 -> Integrator4/1
  TireInertia/1 -> Divide1/2
  Sum/1 -> Divide1/1
  TireFx _r [N]/1 -> Gain/1
  Tb_r [Nm]/1 -> Gain2/1
  Gain/1 -> Sum/2
  Gain2/1 -> Sum/1

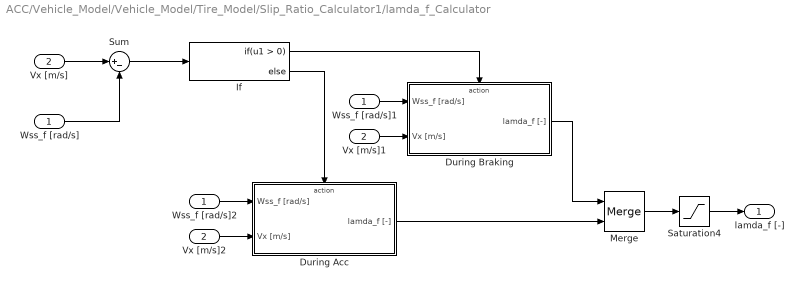
== system ACC/Vehicle_Model/Vehicle_Model/Tire_Model/Slip_Ratio_Calculator1/lamda_f_Calculator ==
  Wss_f [rad/s] : Inport
  Vx [m/s] : Inport  Port=2
  During Acc : Subsystem
  During Braking : Subsystem
  If : If
  Merge : Merge
  Saturation4 : Saturate  UpperLimit=1  LowerLimit=-1
  Sum : Sum  Inputs=|+-
  Vx [m/s]1 : InportShadow  Port=2
  Vx [m/s]2 : InportShadow  Port=2
  Wss_f [rad/s]1 : InportShadow
  Wss_f [rad/s]2 : InportShadow
  lamda_f [-] : Outport
  wires:
  If/1 -> During Braking/Action
  If/2 -> During Acc/Action
  Merge/1 -> Saturation4/1
  During Acc/1(lamda_f [-]) -> Merge/2
  During Braking/1(lamda_f [-]) -> Merge/1
  Wss_f [rad/s]/1 -> Sum/2
  Vx [m/s]/1 -> Sum/1
  Sum/1 -> If/1
  Vx [m/s]1/1 -> During Braking/2(Vx [m/s])
  Wss_f [rad/s]1/1 -> During Braking/1(Wss_f [rad/s])
  Wss_f [rad/s]2/1 -> During Acc/1(Wss_f [rad/s])
  Vx [m/s]2/1 -> During Acc/2(Vx [m/s])
  Saturation4/1 -> lamda_f [-]/1

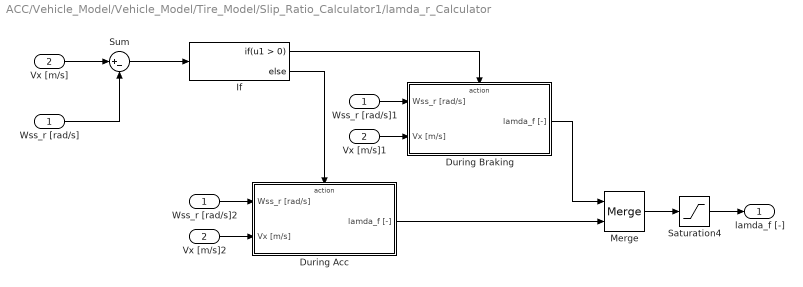
== system ACC/Vehicle_Model/Vehicle_Model/Tire_Model/Slip_Ratio_Calculator1/lamda_r_Calculator ==
  Wss_r [rad/s] : Inport
  Vx [m/s] : Inport  Port=2
  During Acc : Subsystem
  During Braking : Subsystem
  If : If
  Merge : Merge
  Saturation4 : Saturate  UpperLimit=1  LowerLimit=-1
  Sum : Sum  Inputs=|+-
  Vx [m/s]1 : InportShadow  Port=2
  Vx [m/s]2 : InportShadow  Port=2
  Wss_r [rad/s]1 : InportShadow
  Wss_r [rad/s]2 : InportShadow
  lamda_f [-] : Outport
  wires:
  Saturation4/1 -> lamda_f [-]/1
  Vx [m/s]2/1 -> During Acc/2(Vx [m/s])
  Wss_r [rad/s]2/1 -> During Acc/1(Wss_r [rad/s])
  Wss_r [rad/s]1/1 -> During Braking/1(Wss_r [rad/s])
  Vx [m/s]1/1 -> During Braking/2(Vx [m/s])
  Sum/1 -> If/1
  Vx [m/s]/1 -> Sum/1
  Wss_r [rad/s]/1 -> Sum/2
  During Braking/1(lamda_f [-]) -> Merge/1
  During Acc/1(lamda_f [-]) -> Merge/2
  Merge/1 -> Saturation4/1
  If/2 -> During Acc/Action
  If/1 -> During Braking/Action

== system ACC/Vehicle_Model/Vehicle_Model/Tire_Model/Slip_Ratio_Calculator1/lamda_f_Calculator/During Acc ==
  note: (Rw-Vx) / Rw
  note: Slip Ratio During Acc.
  Wss_f [rad/s] : Inport
  Vx [m/s] : Inport  Port=2
  Action Port : ActionPort  ActionType=else
  Divide : Product  Inputs=*/
  Product2 : Product  RndMeth=Zero
  Subtract : Sum  Inputs=-+
  TireRadius : Constant  Value=R_Tire
  lamda_f [-] : Outport
  wires:
  Product2/1 -> Divide/2, Subtract/2
  TireRadius/1 -> Product2/2
  Wss_f [rad/s]/1 -> Product2/1
  Vx [m/s]/1 -> Subtract/1
  Divide/1 -> lamda_f [-]/1
  Subtract/1 -> Divide/1

== system ACC/Vehicle_Model/Vehicle_Model/Tire_Model/Slip_Ratio_Calculator1/lamda_f_Calculator/During Braking ==
  Wss_f [rad/s] : Inport
  Vx [m/s] : Inport  Port=2
  Action Port : ActionPort  ActionType=then
  Divide : Product  Inputs=/*
  Gain : Gain  Gain=-1
  Product2 : Product  RndMeth=Zero
  Subtract : Sum  Inputs=+-
  TireRadius : Constant  Value=R_Tire
  lamda_f [-] : Outport
  wires:
  Vx [m/s]/1 -> Subtract/1, Divide/1
  Wss_f [rad/s]/1 -> Product2/1
  TireRadius/1 -> Product2/2
  Product2/1 -> Subtract/2
  Subtract/1 -> Divide/2
  Divide/1 -> Gain/1
  Gain/1 -> lamda_f [-]/1

== system ACC/Vehicle_Model/Vehicle_Model/Tire_Model/Slip_Ratio_Calculator1/lamda_r_Calculator/During Acc ==
  note: Slip Ratio During Acc.
  note: (Rw-Vx) / Rw
  Wss_r [rad/s] : Inport
  Vx [m/s] : Inport  Port=2
  Action Port : ActionPort  ActionType=else
  Divide : Product  Inputs=*/
  Product2 : Product  RndMeth=Zero
  Subtract : Sum  Inputs=-+
  TireRadius : Constant  Value=R_Tire
  lamda_f [-] : Outport
  wires:
  Subtract/1 -> Divide/1
  Divide/1 -> lamda_f [-]/1
  Vx [m/s]/1 -> Subtract/1
  Wss_r [rad/s]/1 -> Product2/1
  TireRadius/1 -> Product2/2
  Product2/1 -> Subtract/2, Divide/2

== system ACC/Vehicle_Model/Vehicle_Model/Tire_Model/Slip_Ratio_Calculator1/lamda_r_Calculator/During Braking ==
  note: Slip Ratio During Braking
  note: (Rw-Vx) / Vx
  Wss_r [rad/s] : Inport
  Vx [m/s] : Inport  Port=2
  Action Port : ActionPort  ActionType=then
  Divide : Product  Inputs=/*
  Product2 : Product  RndMeth=Zero
  Subtract : Sum  Inputs=-+
  TireRadius : Constant  Value=R_Tire
  lamda_f [-] : Outport
  wires:
  Divide/1 -> lamda_f [-]/1
  Subtract/1 -> Divide/2
  Product2/1 -> Subtract/2
  TireRadius/1 -> Product2/2
  Wss_r [rad/s]/1 -> Product2/1
  Vx [m/s]/1 -> Divide/1, Subtract/1

== stateflow chart ACC/Mode_Selector/Chart ==
  state Cruise_Mode
    du, en : TVSpd = RV+Vx;
    du : send(CruiseFcnCall);
    du : SetSpd = DriverSetSpd;
  state FollowUp_Mode
    du, en : TVSpd = RV+Vx;
    du : send(FollowFcnCall);
    du : SetSpd = TVSpd;
  (default) -> Cruise_Mode
  Cruise_Mode -> FollowUp_Mode : [(RD <= RD_Lower) & (DriverSetSpd >= TVSpd)]
  FollowUp_Mode -> Cruise_Mode : [(RD >RD_Upper) | (DriverSetSpd < TVSpd)]
  data: RD_Upper input; RD_Lower input; RD input; DriverSetSpd input; SetSpd output; Vx input; RV input; TVSpd local
  events: FollowFcnCall output FUNCTION_CALL_EVENT; CruiseFcnCall output FUNCTION_CALL_EVENT
